simulink model "mavsim_chap2"  (R2025b)
settings: Solver=FixedStepDiscrete  StartTime=0.0  StopTime=1000  FixedStep=.1  RelTol=1e-3  EnableMultiTasking=on
InitFcn:
  | addpath('.')
libraries: simulink x6
settings Model: Creator=beard  LastModifiedBy=stutimahajan
settings SolverCC: AlgebraicLoopSolver=TrustRegion
settings DataIOCC: LimitDataPoints=on  SaveFormat=Array  SignalLoggingSaveFormat=ModelDataLogs  ReturnWorkspaceOutputs=off
settings OptimizationCC: ExpressionDepthLimit=2147483647.0  InitFltsAndDblsToZero=on  LifeSpan=inf
settings DebuggingCC: UnderspecifiedInitializationDetection=Classic  MergeDetectMultiDrivingBlocksExec=none  SolverPrmCheckMsg=warning  FcnCallInpInsideContextMsg=warning  UnconnectedInputMsg=warning  UnconnectedOutputMsg=warning  UnconnectedLineMsg=warning  AllowSymbolicDim=off  StateNameClashWarn=warning  SFUnexpectedBacktrackingDiag=warning  SFNoUnconditionalDefaultTransitionDiag=warning  SFExecutionAtInitializationDiag=none  ArithmeticOperatorsInVariantConditions=warning
settings HardwareCC: ProdBitPerPointer=32.0  ProdBitPerSizeT=32.0  ProdBitPerPtrDiffT=32.0  ProdLargestAtomicFloat=None  ProdIntDivRoundTo=Undefined  ProdEndianess=Unspecified  ProdWordSize=32.0  ProdHWDeviceType=32-bit Generic
settings ModelReferenceCC: EnableRefExpFcnMdlSchedulingChecks=on  PropagateSignalLabelsOutOfModel=off
settings SFSimCC: SimUseLocalCustomCode=off  CustomCodeUndefinedFunction=UseInterfaceOnly
settings RTWCC: RTWUseLocalCustomCode=off  GPUComputeCapability=3.5
settings CodeAppCC: StateflowObjectComments=on
settings GRTTargetCC: TargetLangStandard=C89/C90 (ANSI)  CombineOutputUpdateFcns=off  GRTInterface=on
settings ConfigComp: CovMetricSettings=dw  CovSaveCumulativeToWorkspaceVar=on  CovSaveSingleToWorkspaceVar=on  CovExternalEMLEnable=off  CovSFcnEnable=off

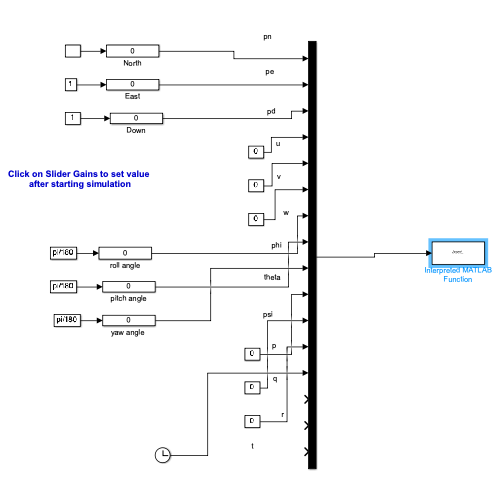
[thumbnail: Simulink's stored preview of the top-level diagram]
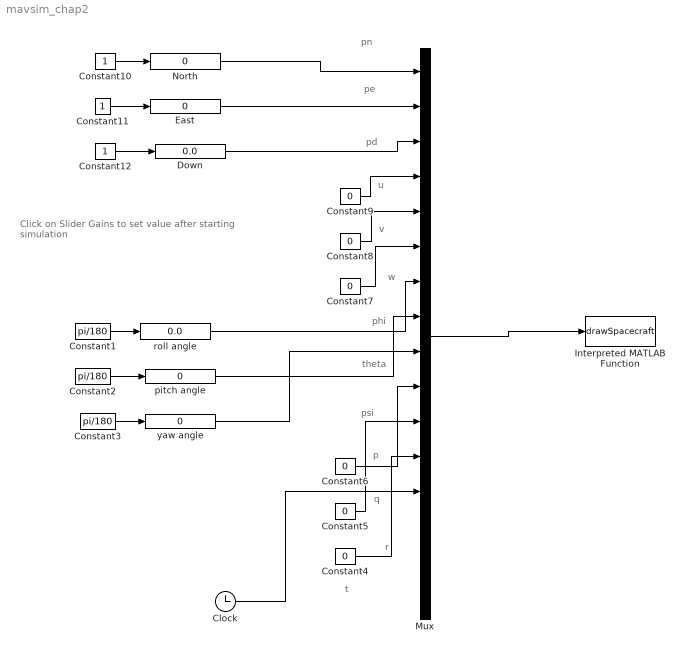
== system mavsim_chap2 ==
  note: t
  note: pn
  note: pe
  note: pd
  note: phi
  note: theta
  note: psi
  note: p
  note: q
  note: r
  note: u
  note: v
  note: w
  note: Click on Slider Gains to set value
      | after starting simulation
  Clock : Clock
  Constant1 : Constant  Value=pi/180
  Constant10 : Constant
  Constant11 : Constant
  Constant12 : Constant
  Constant2 : Constant  Value=pi/180
  Constant3 : Constant  Value=pi/180
  Constant{4..9} (6 alike) : Constant  Value=0
  Down : simulink/Math Operations/Slider Gain  gain=0.0  low=-1000  high=0
  East : simulink/Math Operations/Slider Gain  gain=0  low=-1000  high=1000
  Interpreted MATLAB Function : MATLABFcn  MATLABFcn=drawSpacecraft  OutputDimensions=0
  Mux : Mux  Inputs=16
  North : simulink/Math Operations/Slider Gain  gain=0  low=-900  high=900
  pitch angle : simulink/Math Operations/Slider Gain  gain=0  low=-180  high=180
  roll angle : simulink/Math Operations/Slider Gain  gain=0.0  low=-180  high=180
  "yaw angle " : simulink/Math Operations/Slider Gain  gain=0  low=-180  high=180
  wires:
  Mux/1 -> Interpreted MATLAB Function/1
  roll angle/1 -> Mux/7
  Constant1/1 -> roll angle/1
  pitch angle/1 -> Mux/8
  Constant2/1 -> pitch angle/1
  "yaw angle "/1 -> Mux/9
  Constant3/1 -> "yaw angle "/1
  Constant4/1 -> Mux/12
  Constant5/1 -> Mux/11
  Constant6/1 -> Mux/10
  Constant7/1 -> Mux/6
  Constant8/1 -> Mux/5
  Constant9/1 -> Mux/4
  East/1 -> Mux/2
  Constant11/1 -> East/1
  Down/1 -> Mux/3
  Constant12/1 -> Down/1
  North/1 -> Mux/1
  Constant10/1 -> North/1
  Clock/1 -> Mux/13
